simulink model "ABB_1010"  (R2024a)
settings: Solver=VariableStepAuto  StartTime=0.0  StopTime=200  RelTol=1e-3
model workspace: external: MATLAB File C:\Users\lucas\OneDrive\Documents\MATLAB\projeto final\ABB_1010_DataFile.m (data not in the file)
values from neighbouring files (symbols this model uses):
  g = 9.81    [inicializacaoAntropomorfico.m]
  I1 = [ 0.00243841  0.00000307  0.00007261    [inicializacaoAntropomorfico.m]
  I2 = [ 0.01633569  0.00000387 -0.00034405    [inicializacaoAntropomorfico.m]
  I3 = [ 0.00244760 -0.00000208  0.00000538    [inicializacaoAntropomorfico.m]
  I4 = [ 0.00245792 -0.00000008  0.00003121    [inicializacaoAntropomorfico.m]
  I5 = [ 0.00062165 -0.00000206 -0.00000303    [inicializacaoAntropomorfico.m]
  I6 = [ 0.00000357  0.00000000  0.00000000    [inicializacaoAntropomorfico.m]
  I7 = [(m7*L7^2)/12 0.00000000  0.00000000    [inicializacaoAntropomorfico.m]
  L = [L1, L2, L3, L4, L5, L6, L7]    [inicializacaoAntropomorfico.m]
  Lcm1 = [-0.00258308  0.00024508 -0.01434968]    [inicializacaoAntropomorfico.m]
  Lcm2 = [-0.02078894  0.00020016 -0.10516734]    [inicializacaoAntropomorfico.m]
  Lcm3 = [ 0.00021912  0.00015355 -0.06228290]    [inicializacaoAntropomorfico.m]
  Lcm4 = [-0.00172658 -0.00124140 -0.07369196]    [inicializacaoAntropomorfico.m]
  Lcm5 = [-0.00014110  0.00085992 -0.03825278]    [inicializacaoAntropomorfico.m]
  Lcm6 = [ 0.00002478  0.00000000 -0.00042157]    [inicializacaoAntropomorfico.m]
  Lcm7 = [ 0           0          -0.05000000]    [inicializacaoAntropomorfico.m]
  m = [m1, m2, m3, m4, m5, m6, m7]    [inicializacaoAntropomorfico.m]
  Pf = [  0.05    [inicializacaoAntropomorfico.m]
  Pi = [  0.2    [inicializacaoAntropomorfico.m]
  Raio = [0]    [inicializacaoAntropomorfico.m]
  Sentido = [0]    [inicializacaoAntropomorfico.m]
  Tipo = [1]    [inicializacaoAntropomorfico.m]
undefined symbols (not defined in the file or in its folder): smiData, X, Y, Z
libraries: sm_lib x35, nesl_utility x7
(part 4 of 16)

== matlab function ABB_1010/Cinematica Inversa ==
  data: P input; Qd output; V input; A input; dQd output; d2Qd output; L parameter
function [Qd, dQd, d2Qd] = inversa(P, V, A, L)
    % Entradas:
    % P: Vetor de posição [x, y, z]
    % V: Vetor de velocidades lineares [vx, vy, vz]
    % A: Vetor de acelerações lineares [ax, ay, az]
    % L1, L2: Comprimentos dos elos

    % Saídas:
    % theta: Ângulos articulares [theta1, theta2]
    % thetadot: Velocidades articulares [thetadot1, thetadot2]
    % thetaddot: Acelerações articulares [thetaddot1, thetaddot2]

    % Extrair os valores de P, V e A
    x  = P(1);
    y  = P(2);
    z  = P(3);
    vx = V(1);
    vy = V(2);
    vz = V(3);
    ax = A(1);
    ay = A(2);
    az = A(3);
    
    Lz1 = L(1);
    Lx2 = L(2);
    Lx3 = L(3);
    Lz4 = L(4);
    Lz5 = L(5);
    Lz6 = L(6);

    % Distância radial
    % R  = sqrt(x^2 + y^2);
    % R2 = sqrt(x^2 + (z - Lz1)^2);
    % Ltotal = Lx2 + Lx3 + Lz4  + Lz5 + Lz6;
    % 
    % % Verificação do alcance do manipulador
    % if R >= Ltotal || R2 >= Ltotal
    %     error('O ponto desejado está fora do alcance do manipulador.');
    % end
    % 
    % --- antes de resolver theta2/theta3, troque o bloco radial por:
    theta1 = atan2(y, x);
    
    rho = hypot(x, y);          % robusto para cos(theta1) ~ 0
    r   = hypot(rho, z - Lz1);  % distancia no plano (rho, z-Lz1)
    
    if r < 1e-12
        error('Perto da singularidade do ombro: r ~ 0');
    end
    
    alfa = acos( min(1,max(-1, (r^2 + Lx2^2 - Lx3^2)/(2*Lx2*r) )) );
    beta = atan2(z - Lz1, rho);
    
    cos_phi = (Lx2^2 + Lx3^2 - r^2) / (2*Lx2*Lx3);
    cos_phi = min(1, max(-1, cos_phi));
    sin_phi = sqrt(max(0, 1 - cos_phi^2));
    
    elbow = +1;                         % escolha (+1 cotovelo "down", -1 "up")
    theta2 = beta - elbow*alfa;
    phi    = atan2(elbow*sin_phi, cos_phi);
    theta3 = pi - phi;
    
    % --- substitua seu R06 e a extração do pulso por:
    if ~exist('R06','var') || isempty(R06)
        R06 = eye(3);                   % se não tiver orientação desejada
    end
    
    c1 = cos(theta1);  s1 = sin(theta1);
    c23 = cos(theta2+theta3);  s23 = sin(theta2+theta3);
    
    R03_T = [ c1*c23,  s1*c23, -s23;
             -s1,      c1,      0;
              c1*s23,  s1*s23,  c23];
    
    R36 = R03_T * R06;
    
    sy = hypot(R36(1,3), R36(2,3));
    theta5 = atan2(sy, R36(3,3));
    if sy < 1e-9
        theta4 = 0;
        theta6 = atan2(-R36(1,2), R36(1,1));
    else
        theta4 = atan2(R36(2,3), R36(1,3));
        theta6 = atan2(R36(3,2), -R36(3,1));
    end
    
    Qd = [theta1; theta2; theta3; theta4; theta5; theta6];
    Qd = real(mod(Qd + pi, 2*pi) - pi);

    
    % Jacobiano
    JL = [- Lx3*(cos(theta2)*cos(theta3)*sin(theta1) - sin(theta1)*sin(theta2)*sin(theta3)) - Lz4*(cos(theta4)*(cos(theta2)*cos(theta3)*sin(theta1) - sin(theta1)*sin(theta2)*sin(theta3)) + cos(theta1)*sin(theta4)) - Lz6*(sin(theta5)*(cos(theta4)*(cos(theta2)*cos(theta3)*sin(theta1) - sin(theta1)*sin(theta2)*sin(theta3)) + cos(theta1)*sin(theta4)) + cos(theta5)*(cos(theta2)*sin(theta1)*sin(theta3) + cos(theta3)*sin(theta1)*sin(theta2))) - Lx2*cos(theta2)*sin(theta1),                           -cos(theta1)*(Lx3*sin(theta2 + theta3) + Lx2*sin(theta2) - Lz6*cos(theta2 + theta3)*cos(theta5) + Lz4*sin(theta2 + theta3)*cos(theta4) + Lz6*sin(theta2 + theta3)*cos(theta4)*sin(theta5)), Lz6*cos(theta1)*(cos(theta2 + theta3)*cos(theta5) - sin(theta2 + theta3)*cos(theta4)*sin(theta5)) - Lx3*sin(theta2 + theta3)*cos(theta1) - Lz4*sin(theta2 + theta3)*cos(theta1)*cos(theta4), -(Lz4 + Lz6*sin(theta5))*(cos(theta4)*sin(theta1) + cos(theta1)*cos(theta2)*cos(theta3)*sin(theta4) - cos(theta1)*sin(theta2)*sin(theta3)*sin(theta4)), -Lz6*(sin(theta5)*(cos(theta1)*cos(theta2)*sin(theta3) + cos(theta1)*cos(theta3)*sin(theta2)) - cos(theta5)*(cos(theta4)*(cos(theta1)*cos(theta2)*cos(theta3) - cos(theta1)*sin(theta2)*sin(theta3)) - sin(theta1)*sin(theta4))), 0;
            Lx3*(cos(theta1)*cos(theta2)*cos(theta3) - cos(theta1)*sin(theta2)*sin(theta3)) + Lz4*(cos(theta4)*(cos(theta1)*cos(theta2)*cos(theta3) - cos(theta1)*sin(theta2)*sin(theta3)) - sin(theta1)*sin(theta4)) + Lz6*(cos(theta5)*(cos(theta1)*cos(theta2)*sin(theta3) + cos(theta1)*cos(theta3)*sin(theta2)) + sin(theta5)*(cos(theta4)*(cos(theta1)*cos(theta2)*cos(theta3) - cos(theta1)*sin(theta2)*sin(theta3)) - sin(theta1)*sin(theta4))) + Lx2*cos(theta1)*cos(theta2),                           -sin(theta1)*(Lx3*sin(theta2 + theta3) + Lx2*sin(theta2) - Lz6*cos(theta2 + theta3)*cos(theta5) + Lz4*sin(theta2 + theta3)*cos(theta4) + Lz6*sin(theta2 + theta3)*cos(theta4)*sin(theta5)), Lz6*sin(theta1)*(cos(theta2 + theta3)*cos(theta5) - sin(theta2 + theta3)*cos(theta4)*sin(theta5)) - Lx3*sin(theta2 + theta3)*sin(theta1) - Lz4*sin(theta2 + theta3)*cos(theta4)*sin(theta1),  (Lz4 + Lz6*sin(theta5))*(cos(theta1)*cos(theta4) - cos(theta2)*cos(theta3)*sin(theta1)*sin(theta4) + sin(theta1)*sin(theta2)*sin(theta3)*sin(theta4)), -Lz6*(sin(theta5)*(cos(theta2)*sin(theta1)*sin(theta3) + cos(theta3)*sin(theta1)*sin(theta2)) - cos(theta5)*(cos(theta4)*(cos(theta2)*cos(theta3)*sin(theta1) - sin(theta1)*sin(theta2)*sin(theta3)) + cos(theta1)*sin(theta4))), 0;
                                                                                                                                                                                                                                                                                                                                            0, (Lz6*cos(theta2 + theta3)*sin(theta4 - theta5))/2 - Lx2*cos(theta2) - (Lz6*cos(theta2 + theta3)*sin(theta4 + theta5))/2 - Lz4*cos(theta2 + theta3)*cos(theta4) - Lz6*sin(theta2 + theta3)*cos(theta5) - Lx3*cos(theta2 + theta3),                     - Lx3*cos(theta2 + theta3) - Lz4*cos(theta2 + theta3)*cos(theta4) - Lz6*sin(theta2 + theta3)*cos(theta5) - Lz6*cos(theta2 + theta3)*cos(theta4)*sin(theta5),                                                                   sin(theta2 + theta3)*sin(theta4)*(Lz4 + Lz6*sin(theta5)),                                                                                                - Lz6*cos(theta2 + theta3)*sin(theta5) - Lz6*sin(theta2 + theta3)*cos(theta4)*cos(theta5), 0];
    % 
    % % Verificação da Singularidade do Jacobiano
    % detJ = cos(theta2)*sin(theta3)*sin(theta5)*Lx2^2*Lx3 + cos(theta2)*cos(theta5)*Lx2^2*Lz4*cos(theta3)*cos(theta4)^2 - cos(theta2)*cos(theta5)*Lx2^2*Lz4*cos(theta3) - cos(theta2)*sin(theta3)*sin(theta5)*Lx2^2*Lz4*cos(theta4) - sin(theta2)*sin(theta5)*Lx2*Lx3^2*cos(theta3)^2 - cos(theta2)*sin(theta3)*sin(theta5)*Lx2*Lx3^2*cos(theta3) + sin(theta2)*sin(theta5)*Lx2*Lx3^2 - sin(theta2)*sin(theta5)*Lx2*Lx3*Lz4*cos(theta3)^2*cos(theta4) - cos(theta2)*cos(theta5)*Lx2*Lx3*Lz4*cos(theta3)^2 - cos(theta2)*sin(theta3)*sin(theta5)*Lx2*Lx3*Lz4*cos(theta3)*cos(theta4) + cos(theta5)*sin(theta2)*sin(theta3)*Lx2*Lx3*Lz4*cos(theta3) + cos(theta2)*cos(theta5)*Lx2*Lx3*Lz4*cos(theta4)^2 + sin(theta2)*sin(theta5)*Lx2*Lx3*Lz4*cos(theta4) - cos(theta2)*cos(theta5)*Lx2*Lz4^2*cos(theta3)^2*cos(theta4) + cos(theta5)*sin(theta2)*sin(theta3)*Lx2*Lz4^2*cos(theta3)*cos(theta4) + cos(theta2)*cos(theta5)*Lx2*Lz4^2*cos(theta4);
    % if abs(detJ) < 1e-6
    %     error('Jacobiano próximo de singularidade. Não é possível calcular thetadot.');
    % end
    % 
    lambda2 = 1e-6;
    invJ = JL'/(JL*JL' + lambda2*eye(3));
    
    dtheta1 = dQd(1);
    dtheta2 = dQd(2);
    dtheta3 = dQd(3);
    dtheta4 = dQd(4);
    dtheta5 = dQd(5);
    dtheta6 = dQd(6);
    

    % Derivada do Jacobiano (Jdot)                                                                                                                0,                                                         0, 0, 0];
    dJL = [  dtheta4*(Lz4*(sin(theta4)*(cos(theta2)*cos(theta3)*sin(theta1) - sin(theta1)*sin(theta2)*sin(theta3)) - cos(theta1)*cos(theta4)) + Lz6*sin(theta5)*(sin(theta4)*(cos(theta2)*cos(theta3)*sin(theta1) - sin(theta1)*sin(theta2)*sin(theta3)) - cos(theta1)*cos(theta4))) - dtheta1*(Lx3*(cos(theta1)*cos(theta2)*cos(theta3) - cos(theta1)*sin(theta2)*sin(theta3)) + Lz4*(cos(theta4)*(cos(theta1)*cos(theta2)*cos(theta3) - cos(theta1)*sin(theta2)*sin(theta3)) - sin(theta1)*sin(theta4)) + Lz6*(cos(theta5)*(cos(theta1)*cos(theta2)*sin(theta3) + cos(theta1)*cos(theta3)*sin(theta2)) + sin(theta5)*(cos(theta4)*(cos(theta1)*cos(theta2)*cos(theta3) - cos(theta1)*sin(theta2)*sin(theta3)) - sin(theta1)*sin(theta4))) + Lx2*cos(theta1)*cos(theta2)) + dtheta3*(Lx3*(cos(theta2)*sin(theta1)*sin(theta3) + cos(theta3)*sin(theta1)*sin(theta2)) - Lz6*(cos(theta5)*(cos(theta2)*cos(theta3)*sin(theta1) - sin(theta1)*sin(theta2)*sin(theta3)) - cos(theta4)*sin(theta5)*(cos(theta2)*sin(theta1)*sin(theta3) + cos(theta3)*sin(theta1)*sin(theta2))) + Lz4*cos(theta4)*(cos(theta2)*sin(theta1)*sin(theta3) + cos(theta3)*sin(theta1)*sin(theta2))) + dtheta2*(Lx3*(cos(theta2)*sin(theta1)*sin(theta3) + cos(theta3)*sin(theta1)*sin(theta2)) - Lz6*(cos(theta5)*(cos(theta2)*cos(theta3)*sin(theta1) - sin(theta1)*sin(theta2)*sin(theta3)) - cos(theta4)*sin(theta5)*(cos(theta2)*sin(theta1)*sin(theta3) + cos(theta3)*sin(theta1)*sin(theta2))) + Lx2*sin(theta1)*sin(theta2) + Lz4*cos(theta4)*(cos(theta2)*sin(theta1)*sin(theta3) + cos(theta3)*sin(theta1)*sin(theta2))) + Lz6*dtheta5*(sin(theta5)*(cos(theta2)*sin(theta1)*sin(theta3) + cos(theta3)*sin(theta1)*sin(theta2)) - cos(theta5)*(cos(theta4)*(cos(theta2)*cos(theta3)*sin(theta1) - sin(theta1)*sin(theta2)*sin(theta3)) + cos(theta1)*sin(theta4))), dtheta4*cos(theta1)*(Lz4*sin(theta2 + theta3)*sin(theta4) + Lz6*sin(theta2 + theta3)*sin(theta4)*sin(theta5)) - dtheta5*cos(theta1)*(Lz6*cos(theta2 + theta3)*sin(theta5) + Lz6*sin(theta2 + theta3)*cos(theta4)*cos(theta5)) - dtheta3*cos(theta1)*(Lx3*cos(theta2 + theta3) + Lz4*cos(theta2 + theta3)*cos(theta4) + Lz6*sin(theta2 + theta3)*cos(theta5) + Lz6*cos(theta2 + theta3)*cos(theta4)*sin(theta5)) - dtheta2*cos(theta1)*(Lx3*cos(theta2 + theta3) + Lx2*cos(theta2) + Lz4*cos(theta2 + theta3)*cos(theta4) + Lz6*sin(theta2 + theta3)*cos(theta5) + Lz6*cos(theta2 + theta3)*cos(theta4)*sin(theta5)) + dtheta1*sin(theta1)*(Lx3*sin(theta2 + theta3) + Lx2*sin(theta2) - Lz6*cos(theta2 + theta3)*cos(theta5) + Lz4*sin(theta2 + theta3)*cos(theta4) + Lz6*sin(theta2 + theta3)*cos(theta4)*sin(theta5)), dtheta4*(Lz4*sin(theta2 + theta3)*cos(theta1)*sin(theta4) + Lz6*sin(theta2 + theta3)*cos(theta1)*sin(theta4)*sin(theta5)) + dtheta1*(Lx3*sin(theta2 + theta3)*sin(theta1) - Lz6*sin(theta1)*(cos(theta2 + theta3)*cos(theta5) - sin(theta2 + theta3)*cos(theta4)*sin(theta5)) + Lz4*sin(theta2 + theta3)*cos(theta4)*sin(theta1)) - dtheta2*(Lz6*cos(theta1)*(sin(theta2 + theta3)*cos(theta5) + cos(theta2 + theta3)*cos(theta4)*sin(theta5)) + Lx3*cos(theta2 + theta3)*cos(theta1) + Lz4*cos(theta2 + theta3)*cos(theta1)*cos(theta4)) - dtheta3*(Lz6*cos(theta1)*(sin(theta2 + theta3)*cos(theta5) + cos(theta2 + theta3)*cos(theta4)*sin(theta5)) + Lx3*cos(theta2 + theta3)*cos(theta1) + Lz4*cos(theta2 + theta3)*cos(theta1)*cos(theta4)) - Lz6*dtheta5*cos(theta1)*(cos(theta2 + theta3)*sin(theta5) + sin(theta2 + theta3)*cos(theta4)*cos(theta5)), dtheta4*(Lz4 + Lz6*sin(theta5))*(sin(theta1)*sin(theta4) - cos(theta1)*cos(theta2)*cos(theta3)*cos(theta4) + cos(theta1)*cos(theta4)*sin(theta2)*sin(theta3)) - dtheta1*(Lz4 + Lz6*sin(theta5))*(cos(theta1)*cos(theta4) - cos(theta2)*cos(theta3)*sin(theta1)*sin(theta4) + sin(theta1)*sin(theta2)*sin(theta3)*sin(theta4)) + dtheta2*(cos(theta1)*cos(theta2)*sin(theta3)*sin(theta4) + cos(theta1)*cos(theta3)*sin(theta2)*sin(theta4))*(Lz4 + Lz6*sin(theta5)) + dtheta3*(cos(theta1)*cos(theta2)*sin(theta3)*sin(theta4) + cos(theta1)*cos(theta3)*sin(theta2)*sin(theta4))*(Lz4 + Lz6*sin(theta5)) - Lz6*dtheta5*cos(theta5)*(cos(theta4)*sin(theta1) + cos(theta1)*cos(theta2)*cos(theta3)*sin(theta4) - cos(theta1)*sin(theta2)*sin(theta3)*sin(theta4)),   Lz6*dtheta1*(sin(theta5)*(cos(theta2)*sin(theta1)*sin(theta3) + cos(theta3)*sin(theta1)*sin(theta2)) - cos(theta5)*(cos(theta4)*(cos(theta2)*cos(theta3)*sin(theta1) - sin(theta1)*sin(theta2)*sin(theta3)) + cos(theta1)*sin(theta4))) - Lz6*dtheta2*(sin(theta5)*(cos(theta1)*cos(theta2)*cos(theta3) - cos(theta1)*sin(theta2)*sin(theta3)) + cos(theta4)*cos(theta5)*(cos(theta1)*cos(theta2)*sin(theta3) + cos(theta1)*cos(theta3)*sin(theta2))) - Lz6*dtheta3*(sin(theta5)*(cos(theta1)*cos(theta2)*cos(theta3) - cos(theta1)*sin(theta2)*sin(theta3)) + cos(theta4)*cos(theta5)*(cos(theta1)*cos(theta2)*sin(theta3) + cos(theta1)*cos(theta3)*sin(theta2))) - Lz6*dtheta5*(cos(theta5)*(cos(theta1)*cos(theta2)*sin(theta3) + cos(theta1)*cos(theta3)*sin(theta2)) + sin(theta5)*(cos(theta4)*(cos(theta1)*cos(theta2)*cos(theta3) - cos(theta1)*sin(theta2)*sin(theta3)) - sin(theta1)*sin(theta4))) - Lz6*dtheta4*cos(theta5)*(sin(theta4)*(cos(theta1)*cos(theta2)*cos(theta3) - cos(theta1)*sin(theta2)*sin(theta3)) + cos(theta4)*sin(theta1)), 0;
           - dtheta3*(Lx3*(cos(theta1)*cos(theta2)*sin(theta3) + cos(theta1)*cos(theta3)*sin(theta2)) - Lz6*(cos(theta5)*(cos(theta1)*cos(theta2)*cos(theta3) - cos(theta1)*sin(theta2)*sin(theta3)) - cos(theta4)*sin(theta5)*(cos(theta1)*cos(theta2)*sin(theta3) + cos(theta1)*cos(theta3)*sin(theta2))) + Lz4*cos(theta4)*(cos(theta1)*cos(theta2)*sin(theta3) + cos(theta1)*cos(theta3)*sin(theta2))) - dtheta2*(Lx3*(cos(theta1)*cos(theta2)*sin(theta3) + cos(theta1)*cos(theta3)*sin(theta2)) - Lz6*(cos(theta5)*(cos(theta1)*cos(theta2)*cos(theta3) - cos(theta1)*sin(theta2)*sin(theta3)) - cos(theta4)*sin(theta5)*(cos(theta1)*cos(theta2)*sin(theta3) + cos(theta1)*cos(theta3)*sin(theta2))) + Lx2*cos(theta1)*sin(theta2) + Lz4*cos(theta4)*(cos(theta1)*cos(theta2)*sin(theta3) + cos(theta1)*cos(theta3)*sin(theta2))) - dtheta1*(Lx3*(cos(theta2)*cos(theta3)*sin(theta1) - sin(theta1)*sin(theta2)*sin(theta3)) + Lz4*(cos(theta4)*(cos(theta2)*cos(theta3)*sin(theta1) - sin(theta1)*sin(theta2)*sin(theta3)) + cos(theta1)*sin(theta4)) + Lz6*(sin(theta5)*(cos(theta4)*(cos(theta2)*cos(theta3)*sin(theta1) - sin(theta1)*sin(theta2)*sin(theta3)) + cos(theta1)*sin(theta4)) + cos(theta5)*(cos(theta2)*sin(theta1)*sin(theta3) + cos(theta3)*sin(theta1)*sin(theta2))) + Lx2*cos(theta2)*sin(theta1)) - dtheta4*(Lz4*(sin(theta4)*(cos(theta1)*cos(theta2)*cos(theta3) - cos(theta1)*sin(theta2)*sin(theta3)) + cos(theta4)*sin(theta1)) + Lz6*sin(theta5)*(sin(theta4)*(cos(theta1)*cos(theta2)*cos(theta3) - cos(theta1)*sin(theta2)*sin(theta3)) + cos(theta4)*sin(theta1))) - Lz6*dtheta5*(sin(theta5)*(cos(theta1)*cos(theta2)*sin(theta3) + cos(theta1)*cos(theta3)*sin(theta2)) - cos(theta5)*(cos(theta4)*(cos(theta1)*cos(theta2)*cos(theta3) - cos(theta1)*sin(theta2)*sin(theta3)) - sin(theta1)*sin(theta4))), dtheta4*sin(theta1)*(Lz4*sin(theta2 + theta3)*sin(theta4) + Lz6*sin(theta2 + theta3)*sin(theta4)*sin(theta5)) - dtheta5*sin(theta1)*(Lz6*cos(theta2 + theta3)*sin(theta5) + Lz6*sin(theta2 + theta3)*cos(theta4)*cos(theta5)) - dtheta3*sin(theta1)*(Lx3*cos(theta2 + theta3) + Lz4*cos(theta2 + theta3)*cos(theta4) + Lz6*sin(theta2 + theta3)*cos(theta5) + Lz6*cos(theta2 + theta3)*cos(theta4)*sin(theta5)) - dtheta2*sin(theta1)*(Lx3*cos(theta2 + theta3) + Lx2*cos(theta2) + Lz4*cos(theta2 + theta3)*cos(theta4) + Lz6*sin(theta2 + theta3)*cos(theta5) + Lz6*cos(theta2 + theta3)*cos(theta4)*sin(theta5)) - dtheta1*cos(theta1)*(Lx3*sin(theta2 + theta3) + Lx2*sin(theta2) - Lz6*cos(theta2 + theta3)*cos(theta5) + Lz4*sin(theta2 + theta3)*cos(theta4) + Lz6*sin(theta2 + theta3)*cos(theta4)*sin(theta5)), dtheta4*(Lz4*sin(theta2 + theta3)*sin(theta1)*sin(theta4) + Lz6*sin(theta2 + theta3)*sin(theta1)*sin(theta4)*sin(theta5)) - dtheta2*(Lz6*sin(theta1)*(sin(theta2 + theta3)*cos(theta5) + cos(theta2 + theta3)*cos(theta4)*sin(theta5)) + Lx3*cos(theta2 + theta3)*sin(theta1) + Lz4*cos(theta2 + theta3)*cos(theta4)*sin(theta1)) - dtheta3*(Lz6*sin(theta1)*(sin(theta2 + theta3)*cos(theta5) + cos(theta2 + theta3)*cos(theta4)*sin(theta5)) + Lx3*cos(theta2 + theta3)*sin(theta1) + Lz4*cos(theta2 + theta3)*cos(theta4)*sin(theta1)) - dtheta1*(Lx3*sin(theta2 + theta3)*cos(theta1) - Lz6*cos(theta1)*(cos(theta2 + theta3)*cos(theta5) - sin(theta2 + theta3)*cos(theta4)*sin(theta5)) + Lz4*sin(theta2 + theta3)*cos(theta1)*cos(theta4)) - Lz6*dtheta5*sin(theta1)*(cos(theta2 + theta3)*sin(theta5) + sin(theta2 + theta3)*cos(theta4)*cos(theta5)), dtheta2*(Lz4 + Lz6*sin(theta5))*(cos(theta2)*sin(theta1)*sin(theta3)*sin(theta4) + cos(theta3)*sin(theta1)*sin(theta2)*sin(theta4)) + dtheta3*(Lz4 + Lz6*sin(theta5))*(cos(theta2)*sin(theta1)*sin(theta3)*sin(theta4) + cos(theta3)*sin(theta1)*sin(theta2)*sin(theta4)) - dtheta1*(Lz4 + Lz6*sin(theta5))*(cos(theta4)*sin(theta1) + cos(theta1)*cos(theta2)*cos(theta3)*sin(theta4) - cos(theta1)*sin(theta2)*sin(theta3)*sin(theta4)) - dtheta4*(Lz4 + Lz6*sin(theta5))*(cos(theta1)*sin(theta4) + cos(theta2)*cos(theta3)*cos(theta4)*sin(theta1) - cos(theta4)*sin(theta1)*sin(theta2)*sin(theta3)) + Lz6*dtheta5*cos(theta5)*(cos(theta1)*cos(theta4) - cos(theta2)*cos(theta3)*sin(theta1)*sin(theta4) + sin(theta1)*sin(theta2)*sin(theta3)*sin(theta4)), - Lz6*dtheta5*(sin(theta5)*(cos(theta4)*(cos(theta2)*cos(theta3)*sin(theta1) - sin(theta1)*sin(theta2)*sin(theta3)) + cos(theta1)*sin(theta4)) + cos(theta5)*(cos(theta2)*sin(theta1)*sin(theta3) + cos(theta3)*sin(theta1)*sin(theta2))) - Lz6*dtheta2*(sin(theta5)*(cos(theta2)*cos(theta3)*sin(theta1) - sin(theta1)*sin(theta2)*sin(theta3)) + cos(theta4)*cos(theta5)*(cos(theta2)*sin(theta1)*sin(theta3) + cos(theta3)*sin(theta1)*sin(theta2))) - Lz6*dtheta3*(sin(theta5)*(cos(theta2)*cos(theta3)*sin(theta1) - sin(theta1)*sin(theta2)*sin(theta3)) + cos(theta4)*cos(theta5)*(cos(theta2)*sin(theta1)*sin(theta3) + cos(theta3)*sin(theta1)*sin(theta2))) - Lz6*dtheta1*(sin(theta5)*(cos(theta1)*cos(theta2)*sin(theta3) + cos(theta1)*cos(theta3)*sin(theta2)) - cos(theta5)*(cos(theta4)*(cos(theta1)*cos(theta2)*cos(theta3) - cos(theta1)*sin(theta2)*sin(theta3)) - sin(theta1)*sin(theta4))) - Lz6*dtheta4*cos(theta5)*(sin(theta4)*(cos(theta2)*cos(theta3)*sin(theta1) - sin(theta1)*sin(theta2)*sin(theta3)) - cos(theta1)*cos(theta4)), 0;
                                                                                                                                                                                                                                                                                                                                                                                                                                                                                                                                                                                                                                                                                                                                                                                                                                                                                                                                                                                                                                                                                                                                                                                                                                                                                             0,                     dtheta4*((Lz6*cos(theta2 + theta3)*cos(theta4 - theta5))/2 - (Lz6*cos(theta2 + theta3)*cos(theta4 + theta5))/2 + Lz4*cos(theta2 + theta3)*sin(theta4)) - dtheta5*((Lz6*cos(theta2 + theta3)*cos(theta4 + theta5))/2 + (Lz6*cos(theta2 + theta3)*cos(theta4 - theta5))/2 - Lz6*sin(theta2 + theta3)*sin(theta5)) + dtheta3*(Lx3*sin(theta2 + theta3) + (Lz6*sin(theta2 + theta3)*sin(theta4 + theta5))/2 - Lz6*cos(theta2 + theta3)*cos(theta5) + Lz4*sin(theta2 + theta3)*cos(theta4) - (Lz6*sin(theta2 + theta3)*sin(theta4 - theta5))/2) + dtheta2*(Lx3*sin(theta2 + theta3) + Lx2*sin(theta2) + (Lz6*sin(theta2 + theta3)*sin(theta4 + theta5))/2 - Lz6*cos(theta2 + theta3)*cos(theta5) + Lz4*sin(theta2 + theta3)*cos(theta4) - (Lz6*sin(theta2 + theta3)*sin(theta4 - theta5))/2),                                                                                                                                                                                                         dtheta2*(Lx3*sin(theta2 + theta3) - Lz6*cos(theta2 + theta3)*cos(theta5) + Lz4*sin(theta2 + theta3)*cos(theta4) + Lz6*sin(theta2 + theta3)*cos(theta4)*sin(theta5)) + dtheta3*(Lx3*sin(theta2 + theta3) - Lz6*cos(theta2 + theta3)*cos(theta5) + Lz4*sin(theta2 + theta3)*cos(theta4) + Lz6*sin(theta2 + theta3)*cos(theta4)*sin(theta5)) + dtheta5*(Lz6*sin(theta2 + theta3)*sin(theta5) - Lz6*cos(theta2 + theta3)*cos(theta4)*cos(theta5)) + dtheta4*(Lz4*cos(theta2 + theta3)*sin(theta4) + Lz6*cos(theta2 + theta3)*sin(theta4)*sin(theta5)),                                                                                                                                                                                                                                                                                                                                                 dtheta2*cos(theta2 + theta3)*sin(theta4)*(Lz4 + Lz6*sin(theta5)) + dtheta3*cos(theta2 + theta3)*sin(theta4)*(Lz4 + Lz6*sin(theta5)) + dtheta4*sin(theta2 + theta3)*cos(theta4)*(Lz4 + Lz6*sin(theta5)) + Lz6*dtheta5*sin(theta2 + theta3)*cos(theta5)*sin(theta4),                                                                                                                                                                                                                                                                                                                                                                                                                                                                                  dtheta2*(Lz6*sin(theta2 + theta3)*sin(theta5) - Lz6*cos(theta2 + theta3)*cos(theta4)*cos(theta5)) + dtheta3*(Lz6*sin(theta2 + theta3)*sin(theta5) - Lz6*cos(theta2 + theta3)*cos(theta4)*cos(theta5)) - dtheta5*(Lz6*cos(theta2 + theta3)*cos(theta5) - Lz6*sin(theta2 + theta3)*cos(theta4)*sin(theta5)) + Lz6*dtheta4*sin(theta2 + theta3)*cos(theta5)*sin(theta4), 0];
 
    dQd  = invJ * [vx; vy; vz];
    d2Qd = invJ * ( [ax; ay; az] - dJL * dQd );
end
